simulink model "Three_Step_DTZNN"  (R2024a)
settings: Solver=ode1  StartTime=0.0  StopTime=10.0  FixedStep=0.01  RelTol=1e-3
values from neighbouring files (symbols this model uses):
  gamma = 1.0    (= 1)    [ctznn.m]    (also in setup.m = 40)
  tau = 0.01    [setup.m]
  X0 = rand(4,1)*2-1    [ctznn.m]    (also in setup.m = eye(2))
  X1 = X0 - tau*X0*dA(0)*X0 - h*X0*(A(0)*X0-eye(2))    [setup.m]
  X2 = X1 - tau*X1*dA(1*tau)*X1 - h*X1*(A(1*tau)*X1-eye(2))    [setup.m]
settings Model: Creator=uli_2  LastModifiedBy=uli_2
settings DebuggingCC: UnconnectedInputMsg=warning  UnconnectedOutputMsg=warning  UnconnectedLineMsg=warning
settings ModelReferenceCC: EnableRefExpFcnMdlSchedulingChecks=on
settings RTWCC: GPUComputeCapability=3.5  DLArmComputeVersion=19.05

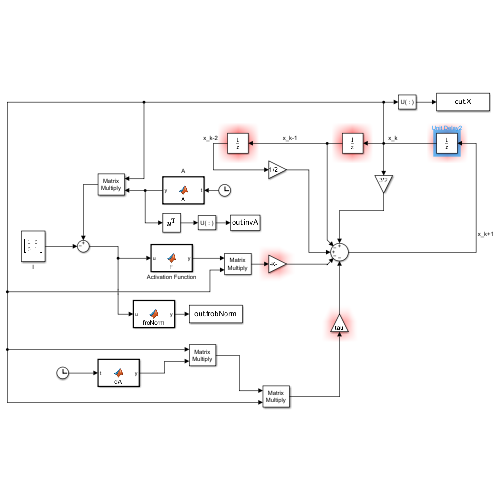
[thumbnail: Simulink's stored preview of the top-level diagram]
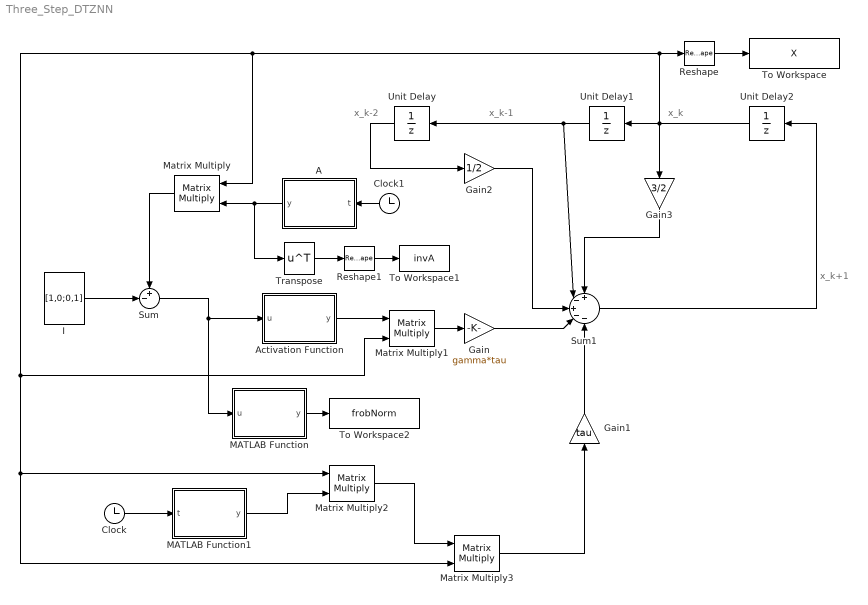
== system Three_Step_DTZNN ==
  note: x_k+1
  note: x_k-2
  note: x_k-1
  note: x_k
  A : MATLAB Function  TreatAsAtomicUnit=on
  Activation Function : MATLAB Function  TreatAsAtomicUnit=on
  Clock : Clock
  Clock1 : Clock
  Gain : Gain  Gain=gamma*tau
  Gain1 : Gain  Gain=tau
  Gain2 : Gain  Gain=1/2
  Gain3 : Gain  Gain=3/2
  I : Constant  Value=[1,0;0,1]
  MATLAB Function : MATLAB Function  TreatAsAtomicUnit=on
  MATLAB Function1 : MATLAB Function  TreatAsAtomicUnit=on
  Matrix Multiply{,1..3} (4 alike) : Product  Multiplication=Matrix(*)
  Reshape : Reshape
  Reshape1 : Reshape
  Sum : Sum  Inputs=+-|
  Sum1 : Sum  Inputs=+-+--
  To Workspace : ToWorkspace  VariableName=X  SaveFormat=Timeseries  SampleTime=-1
  To Workspace1 : ToWorkspace  VariableName=invA  SaveFormat=Timeseries  SampleTime=-1
  To Workspace2 : ToWorkspace  VariableName=frobNorm  SaveFormat=Timeseries  SampleTime=-1
  Transpose : Math  Operator=transpose
  Unit Delay : UnitDelay  InitialCondition=X0  SampleTime=-1  HasFrameUpgradeWarning=on
  Unit Delay1 : UnitDelay  InitialCondition=X1  SampleTime=-1  HasFrameUpgradeWarning=on
  Unit Delay2 : UnitDelay  InitialCondition=X2  SampleTime=-1  HasFrameUpgradeWarning=on
  wires:
  Clock/1 -> MATLAB Function1/1(t)
  Clock1/1 -> A/1(t)
  Matrix Multiply3/1 -> Gain1/1
  Matrix Multiply2/1 -> Matrix Multiply3/1
  Matrix Multiply/1 -> Sum/1
  Sum/1 -> MATLAB Function/1(u), Activation Function/1(u)
  Sum1/1 -> Unit Delay2/1
  Transpose/1 -> Reshape1/1
  Activation Function/1(y) -> Matrix Multiply1/1
  MATLAB Function1/1(y) -> Matrix Multiply2/2
  Matrix Multiply1/1 -> Gain/1
  I/1 -> Sum/2
  A/1(y) -> Transpose/1, Matrix Multiply/2
  Unit Delay/1 -> Gain2/1
  Unit Delay2/1 -> Gain3/1, Reshape/1, Matrix Multiply/1, Matrix Multiply1/2, Matrix Multiply3/2, Matrix Multiply2/1, Unit Delay1/1
  Unit Delay1/1 -> Unit Delay/1, Sum1/2
  Gain1/1 -> Sum1/5
  Gain/1 -> Sum1/4
  Gain2/1 -> Sum1/3
  Gain3/1 -> Sum1/1
  MATLAB Function/1(y) -> To Workspace2/1
  Reshape/1 -> To Workspace/1
  Reshape1/1 -> To Workspace1/1

== matlab function Three_Step_DTZNN/A ==
  data: t input; y output
function y = A(t)

y = [sin(t), cos(t); -cos(t), sin(t)];

== matlab function Three_Step_DTZNN/Activation Function ==
  data: u input; y output
function y = F(u)
    y = u;
%     p = 3; zeta = 4;
%     if abs(u) >= 1
%         y = u.^p;
%     else
%         y = ((1+exp(-zeta))/(1-exp(-zeta)) * (1-exp(-zeta*u))./(1+exp(-zeta*u)));
%     end

== matlab function Three_Step_DTZNN/MATLAB Function ==
  data: u input; y output
function y = froNorm(u)
    y = norm(u, 'fro');

== matlab function Three_Step_DTZNN/MATLAB Function1 ==
  data: t input; y output
function y = dA(t)

y = [cos(t), -sin(t); sin(t), cos(t)];
